simulink model "quad_model_linear"  (R2026a)
settings: Solver=ode4  FixedStep=0.01
values from neighbouring files (symbols this model uses):
  A_lin = lm.A    [setup_quad_linear.m]
  B_lin = lm.B    [setup_quad_linear.m]
  dx0_lin = x_ic - x0_lin    [setup_quad_linear.m]
  u0_lin = lm.u0    [setup_quad_linear.m]
  x0_lin = lm.x0    [setup_quad_linear.m]
settings Model: Creator=graest  LastModifiedBy=graest

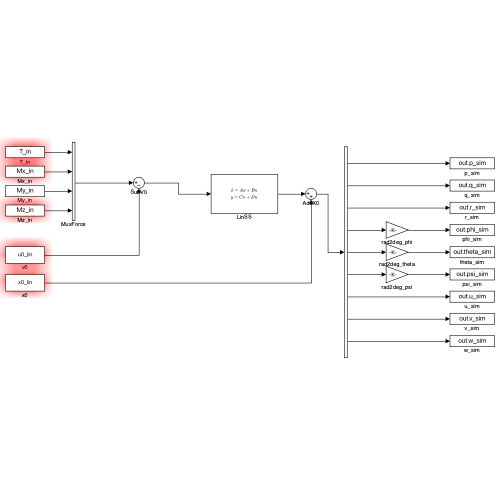
[thumbnail: Simulink's stored preview of the top-level diagram]
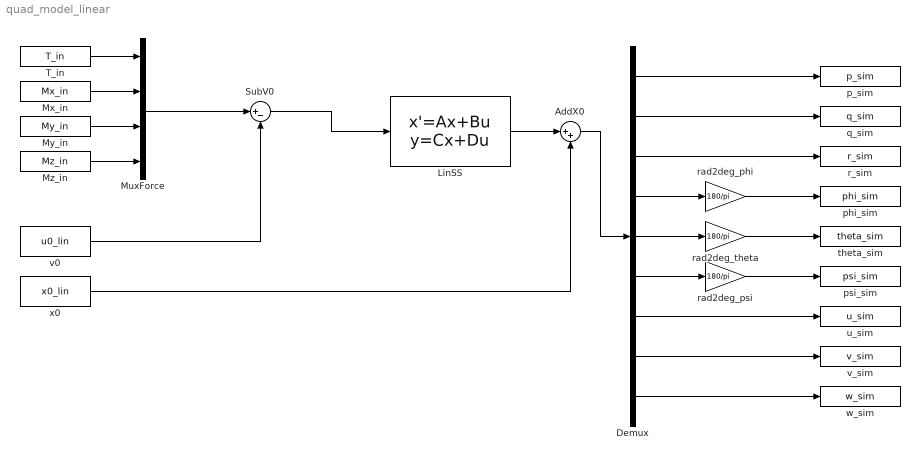
== system quad_model_linear ==
  AddX0 : Sum  Inputs=|++
  Demux : Demux  Outputs=9
  LinSS : StateSpace  A=A_lin  B=B_lin  C=eye(9)  D=zeros(9,4)  InitialCondition=dx0_lin
  MuxForce : Mux
  Mx_in : FromWorkspace  VariableName=Mx_in
  My_in : FromWorkspace  VariableName=My_in
  Mz_in : FromWorkspace  VariableName=Mz_in
  SubV0 : Sum  Inputs=|+-
  T_in : FromWorkspace  VariableName=T_in
  p_sim : ToWorkspace  VariableName=p_sim  SaveFormat=Timeseries  SampleTime=-1
  phi_sim : ToWorkspace  VariableName=phi_sim  SaveFormat=Timeseries  SampleTime=-1
  psi_sim : ToWorkspace  VariableName=psi_sim  SaveFormat=Timeseries  SampleTime=-1
  q_sim : ToWorkspace  VariableName=q_sim  SaveFormat=Timeseries  SampleTime=-1
  r_sim : ToWorkspace  VariableName=r_sim  SaveFormat=Timeseries  SampleTime=-1
  rad2deg_phi : Gain  Gain=180/pi
  rad2deg_psi : Gain  Gain=180/pi
  rad2deg_theta : Gain  Gain=180/pi
  theta_sim : ToWorkspace  VariableName=theta_sim  SaveFormat=Timeseries  SampleTime=-1
  u_sim : ToWorkspace  VariableName=u_sim  SaveFormat=Timeseries  SampleTime=-1
  v0 : Constant  Value=u0_lin
  v_sim : ToWorkspace  VariableName=v_sim  SaveFormat=Timeseries  SampleTime=-1
  w_sim : ToWorkspace  VariableName=w_sim  SaveFormat=Timeseries  SampleTime=-1
  x0 : Constant  Value=x0_lin
  wires:
  T_in/1 -> MuxForce/1
  Mx_in/1 -> MuxForce/2
  My_in/1 -> MuxForce/3
  Mz_in/1 -> MuxForce/4
  MuxForce/1 -> SubV0/1
  v0/1 -> SubV0/2
  SubV0/1 -> LinSS/1
  LinSS/1 -> AddX0/1
  x0/1 -> AddX0/2
  AddX0/1 -> Demux/1
  Demux/1 -> p_sim/1
  Demux/2 -> q_sim/1
  Demux/3 -> r_sim/1
  Demux/7 -> u_sim/1
  Demux/8 -> v_sim/1
  Demux/9 -> w_sim/1
  Demux/4 -> rad2deg_phi/1
  Demux/5 -> rad2deg_theta/1
  Demux/6 -> rad2deg_psi/1
  rad2deg_phi/1 -> phi_sim/1
  rad2deg_theta/1 -> theta_sim/1
  rad2deg_psi/1 -> psi_sim/1
